simulink subsystem "rss_inverter_model"  (R2023a)
settings: Solver=VariableStepAuto  StartTime=0.0  StopTime=10.0  RelTol=1e-3
undefined symbols (not defined in the file): Down, parPwmSwtcFreq, parPwmSwtcFreq_u16n0b0, Up
libraries: eePwmGenerator x3, PELOPWM02MSEREF x3, autolibinverter x1, PEB601MSEREF x1, mcbplantlib x1
settings Model: Creator=CAV2OFO  LastModifiedBy=lenovo
settings SolverCC: AlgebraicLoopSolver=TrustRegion
settings OptimizationCC: ReuseModelBlockBuffer=off
settings DebuggingCC: UnconnectedInputMsg=warning  UnconnectedOutputMsg=warning  UnconnectedLineMsg=warning
settings ModelReferenceCC: EnableRefExpFcnMdlSchedulingChecks=on
settings RTWCC: DLArmComputeVersion=19.05

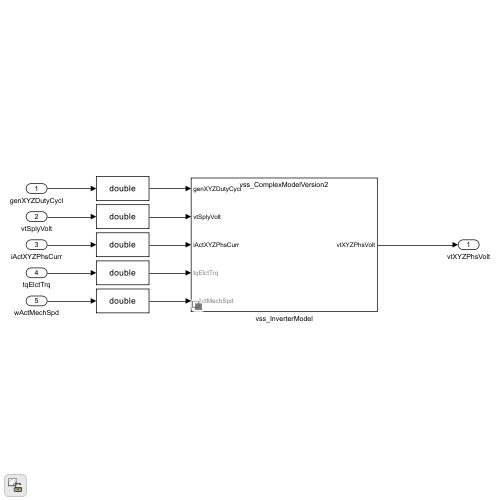
[thumbnail: Simulink's stored preview of the top-level diagram]
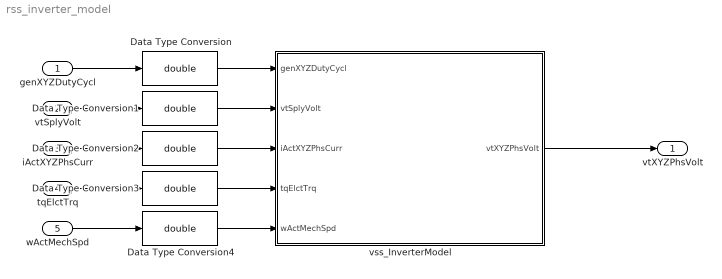
== system rss_inverter_model ==
  genXYZDutyCycl : Inport
  vtSplyVolt : Inport  Port=2
  iActXYZPhsCurr : Inport  Port=3
  tqElctTrq : Inport  Port=4
  wActMechSpd : Inport  Port=5
  Data Type Conversion{,1..4} (5 alike) : DataTypeConversion  OutDataTypeStr=double  SaturateOnIntegerOverflow=off  RndMeth=Floor
  vss_InverterModel : Subsystem  Variant=on  VariantControlMode=label  LabelModeActiveChoice=parCompMdlVrs2
  vtXYZPhsVolt : Outport
  wires:
  genXYZDutyCycl/1 -> Data Type Conversion/1
  vss_InverterModel/1(vtXYZPhsVolt) -> vtXYZPhsVolt/1
  vtSplyVolt/1 -> Data Type Conversion1/1
  iActXYZPhsCurr/1 -> Data Type Conversion2/1
  tqElctTrq/1 -> Data Type Conversion3/1
  wActMechSpd/1 -> Data Type Conversion4/1
  Data Type Conversion/1 -> vss_InverterModel/1(genXYZDutyCycl)
  Data Type Conversion1/1 -> vss_InverterModel/2(vtSplyVolt)
  Data Type Conversion2/1 -> vss_InverterModel/3(iActXYZPhsCurr)
  Data Type Conversion3/1 -> vss_InverterModel/4(tqElctTrq)
  Data Type Conversion4/1 -> vss_InverterModel/5(wActMechSpd)

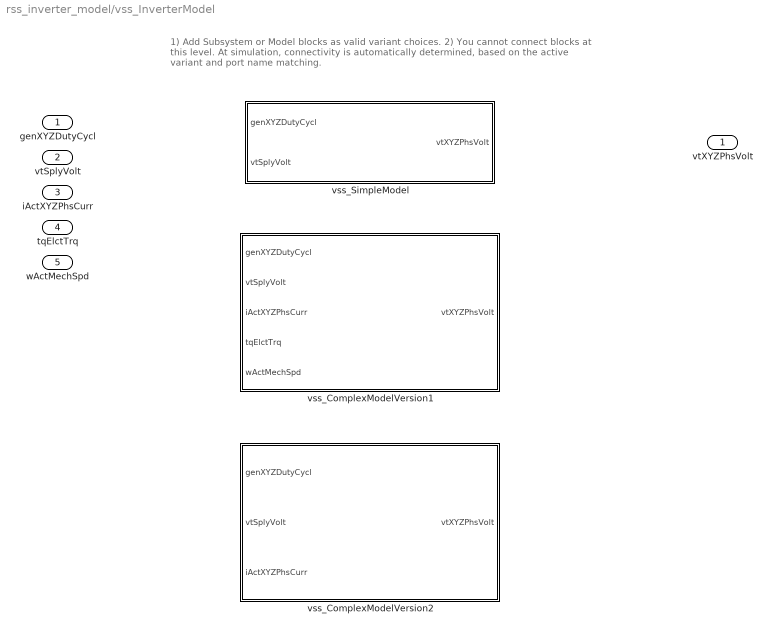
== system rss_inverter_model/vss_InverterModel ==
  note: 1) Add Subsystem or Model blocks as valid variant choices.
      | 2) You cannot connect blocks at this level. At simulation, connectivity is automatically
      | determined, based on the active variant and port name matching.
  genXYZDutyCycl : Inport
  vtSplyVolt : Inport  Port=2
  iActXYZPhsCurr : Inport  Port=3
  tqElctTrq : Inport  Port=4
  wActMechSpd : Inport  Port=5
  vss_ComplexModelVersion1 : Subsystem  VariantControl=parCompMdlVrs1
  vss_ComplexModelVersion2 : Subsystem  VariantControl=parCompMdlVrs2
  vss_SimpleModel : Subsystem  VariantControl=parSmplMdl
  vtXYZPhsVolt : Outport

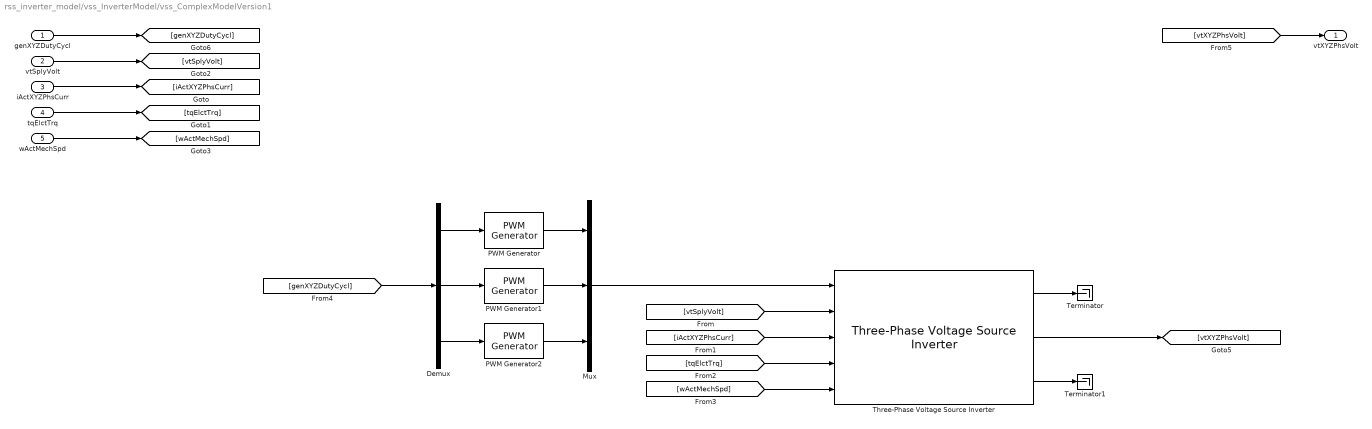
== system rss_inverter_model/vss_InverterModel/vss_ComplexModelVersion1 ==
  genXYZDutyCycl : Inport
  vtSplyVolt : Inport  Port=2
  iActXYZPhsCurr : Inport  Port=3
  tqElctTrq : Inport  Port=4
  wActMechSpd : Inport  Port=5
  Demux : Demux  Outputs=3
  Mux : Mux  Inputs=3
  PWM Generator : eePwmGenerator/PWM Generator  CarrCount=Up-Down  Tper=1/double(parPwmSwtcFreq_u16n0b0)  Tdelay=0  Ts=1/double(parPwmSwtcFreq_u16n0b0)/10
  PWM Generator1 : eePwmGenerator/PWM Generator  CarrCount=Up-Down  Tper=1/double(parPwmSwtcFreq_u16n0b0)  Tdelay=0  Ts=1/double(parPwmSwtcFreq_u16n0b0)/10
  PWM Generator2 : eePwmGenerator/PWM Generator  CarrCount=Up-Down  Tper=1/double(parPwmSwtcFreq_u16n0b0)  Tdelay=0  Ts=1/double(parPwmSwtcFreq_u16n0b0)/10
  Terminator : Terminator
  Terminator1 : Terminator
  Three-Phase Voltage Source Inverter : autolibinverter/Three-Phase Voltage Source Inverter  InvrtrTmpInpEnbl=off  enable_hdl=off  model_type=Switch inputs  fs=10000  w_eff_bp=[-1000 -500 0 500 1000]  n1=128  T_eff_bp=[-200 -100 0 100 200]  Temp_eff_bp=[213.15 293.15 373.15]  n2=128  ploss_table=[0 0 0 0 0;0 0 0 0 0;0 0 0 0 0;0 0 0 0 0;0 0 0 0 0]  ploss_table_3d=cat(3,0.95*[1 0.999 0.989 0.997 0.996;0.995 0.994 0.993 0.992 0.991;0.990 0.989 0.988 0.987 0.986;0.985 0.984 0.983 0.982 0.981;0.980 0.979 0.978 0.977 0.976],[1 0.999 0.989 0.997 0.996;0.995 0.994 0.993 0.992 0.991;0.990 0.989 0.988 0.987 0.986;0.985 0.984 0.983 0.982 0.981;0.980 0.979 0.978 0.977 0.976],0.92*[1 0.999 0.989 0.997 0.996;0.995 0.994 0.993 0.992 0.991;0.990 0.989 0.988 0.987 0.986;0.985 0.984 0.983 0.982 0.981;0.980 0.979 0.978 0.977 0.976])  preExtrapFlag=off  u1max=1000  u1min=-1000  u2max=200  u2min=-200  intPrec=23  RefBlkName='autolibmappedmotor/Mapped Motor'  CalLossMapData={}  CalLossWithTempMapData={}
  vtXYZPhsVolt : Outport
  wires:
  Three-Phase Voltage Source Inverter/3 -> Terminator1/1
  Demux/1 -> PWM Generator/1
  PWM Generator1/1 -> Mux/2
  iActXYZPhsCurr/1 -> [iActXYZPhsCurr]
  PWM Generator2/1 -> Mux/3
  Demux/3 -> PWM Generator2/1
  Three-Phase Voltage Source Inverter/2 -> [vtXYZPhsVolt]
  PWM Generator/1 -> Mux/1
  [iActXYZPhsCurr] -> Three-Phase Voltage Source Inverter/3
  [vtXYZPhsVolt] -> vtXYZPhsVolt/1
  Demux/2 -> PWM Generator1/1
  [vtSplyVolt] -> Three-Phase Voltage Source Inverter/2
  wActMechSpd/1 -> [wActMechSpd]
  Mux/1 -> Three-Phase Voltage Source Inverter/1
  vtSplyVolt/1 -> [vtSplyVolt]
  Three-Phase Voltage Source Inverter/1 -> Terminator/1
  genXYZDutyCycl/1 -> [genXYZDutyCycl]
  [wActMechSpd] -> Three-Phase Voltage Source Inverter/5
  [genXYZDutyCycl] -> Demux/1
  tqElctTrq/1 -> [tqElctTrq]
  [tqElctTrq] -> Three-Phase Voltage Source Inverter/4

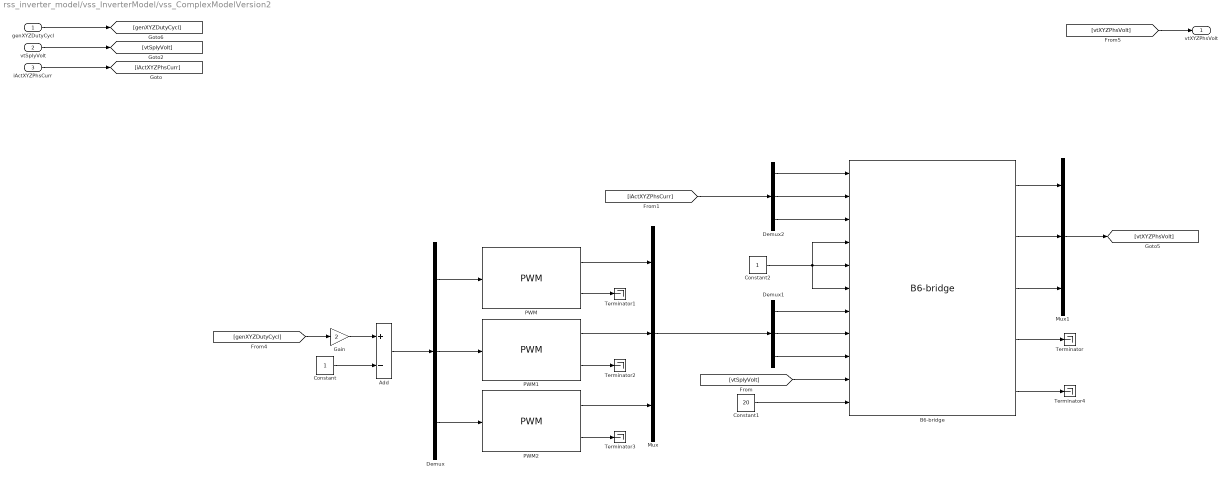
== system rss_inverter_model/vss_InverterModel/vss_ComplexModelVersion2 ==
  genXYZDutyCycl : Inport
  vtSplyVolt : Inport  Port=2
  iActXYZPhsCurr : Inport  Port=3
  Add : Sum  Inputs=+-
  B6-bridge : PEB601MSEREF/B6-bridge  Tag=PEB601MSEREF  RT20=1e-3  RD20=1e-3  VT20=0  VD20=0.7  IGBT=off  Ieps=1e-3  alphaRT=0  alphaRD=0  alphaVT=0  alphaVD=0
      settings: AttributesFormatString=<%<Tag>>
  Constant : Constant
  Constant1 : Constant  Value=20
  Constant2 : Constant
  Demux : Demux  Outputs=3
  Demux1 : Demux  Outputs=3
  Demux2 : Demux  Outputs=3
  Gain : Gain  Gain=2
  Mux : Mux  Inputs=3
  Mux1 : Mux  Inputs=3
  PWM : PELOPWM02MSEREF/PWM  Tag=PELOPWM02MSEREF  mode=middle centered  Tpl=1/parPwmSwtcFreq  disc=off  off=on  Td=6.25e-6
      settings: AttributesFormatString=<%<Tag>>
  PWM1 : PELOPWM02MSEREF/PWM  Tag=PELOPWM02MSEREF  mode=middle centered  Tpl=1/parPwmSwtcFreq  disc=off  off=on  Td=6.25e-6
      settings: AttributesFormatString=<%<Tag>>
  PWM2 : PELOPWM02MSEREF/PWM  Tag=PELOPWM02MSEREF  mode=middle centered  Tpl=1/parPwmSwtcFreq  disc=off  off=on  Td=6.25e-6
      settings: AttributesFormatString=<%<Tag>>
  Terminator{,1..4} (5 alike) : Terminator
  vtXYZPhsVolt : Outport
  wires:
  Mux1/1 -> [vtXYZPhsVolt]
  B6-bridge/3 -> Mux1/3
  B6-bridge/1 -> Mux1/1
  B6-bridge/2 -> Mux1/2
  B6-bridge/5 -> Terminator4/1
  B6-bridge/4 -> Terminator/1
  Constant2/1 -> B6-bridge/5, B6-bridge/4, B6-bridge/6
  Constant1/1 -> B6-bridge/11
  [iActXYZPhsCurr] -> Demux2/1
  Demux2/2 -> B6-bridge/2
  Demux2/3 -> B6-bridge/3
  Demux2/1 -> B6-bridge/1
  Mux/1 -> Demux1/1
  Demux1/3 -> B6-bridge/9
  Demux1/2 -> B6-bridge/8
  Demux1/1 -> B6-bridge/7
  [vtSplyVolt] -> B6-bridge/10
  PWM2/1 -> Mux/3
  PWM1/1 -> Mux/2
  PWM/1 -> Mux/1
  PWM2/2 -> Terminator3/1
  PWM1/2 -> Terminator2/1
  PWM/2 -> Terminator1/1
  Demux/3 -> PWM2/1
  Add/1 -> Demux/1
  Demux/1 -> PWM/1
  Demux/2 -> PWM1/1
  Constant/1 -> Add/2
  Gain/1 -> Add/1
  [genXYZDutyCycl] -> Gain/1
  iActXYZPhsCurr/1 -> [iActXYZPhsCurr]
  [vtXYZPhsVolt] -> vtXYZPhsVolt/1
  vtSplyVolt/1 -> [vtSplyVolt]
  genXYZDutyCycl/1 -> [genXYZDutyCycl]

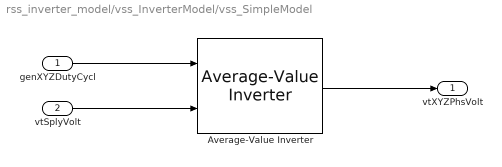
== system rss_inverter_model/vss_InverterModel/vss_SimpleModel ==
  genXYZDutyCycl : Inport
  vtSplyVolt : Inport  Port=2
  Average-Value Inverter : mcbplantlib/Average-Value Inverter
  vtXYZPhsVolt : Outport
  wires:
  Average-Value Inverter/1 -> vtXYZPhsVolt/1
  genXYZDutyCycl/1 -> Average-Value Inverter/1
  vtSplyVolt/1 -> Average-Value Inverter/2
